simulink model "m02_simulate"  (R2024b)
settings: Solver=VariableStepAuto  StartTime=0.0  StopTime=Tsim  RelTol=1e-3
model workspace (MAT data in the model file):
  C_3 = 1e-07
  Cin_2 = 0.0001
  Cout_2 = 0.0001
  Goff_2 = 1e-06
  L_3 = 0.000277
  L_4 = 0.001
  Len_3 = 1
  Lt_2 = 3.042e-05
  N_2 = 1
  R_1 = 1
  R_3 = 1
  R_c_3 = 1e-06
  Rds_2 = 1e-06
  Rt_2 = 0.001
  Tsim = 0.01
  Tstep = 1e-05
  Vf_2 = 0.001
  fs_2 = 5000
libraries: nesl_utility x7, fl_lib x4, ODEsim x4
settings Model: Creator=cao2851  LastModifiedBy=cao2851
settings DataIOCC: ExternalInput=ds{1}  LoadExternalInput=on

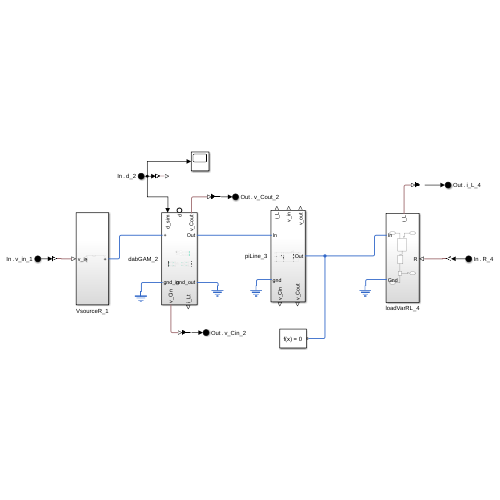
[thumbnail: Simulink's stored preview of the top-level diagram]
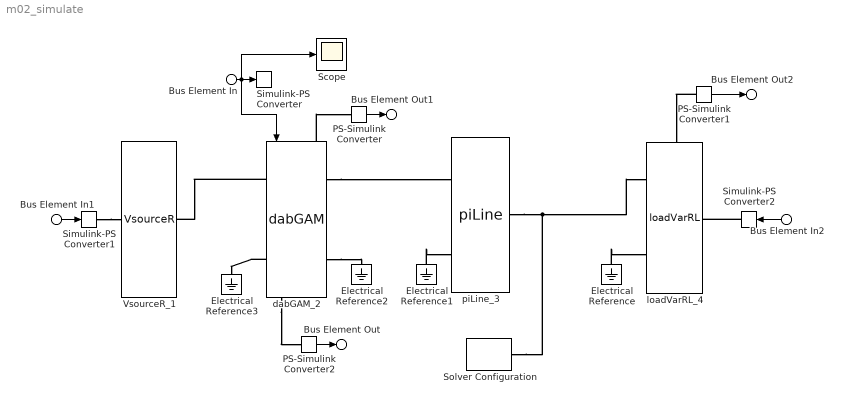
== system m02_simulate ==
  Bus Element In : Inport  PortName=In  Element=d_2
  Bus Element In1 : Inport  PortName=In  Element=v_in_1
  Bus Element In2 : Inport  PortName=In  Element=R_4
  Electrical Reference{,1..3} (4 alike) : fl_lib/Electrical/Electrical Elements/Electrical Reference
  PS-Simulink Converter : nesl_utility/PS-Simulink Converter  PhysicalDomain=network_engine_domain  SubClassName=ps_output  LeftPortType=input  RightPortType=output  PseudoPeriodic=off  Frequencies=[]  VectorFormat=inherit  Unit=inherit  AffineConversion=off
  PS-Simulink Converter1 : nesl_utility/PS-Simulink Converter  PhysicalDomain=network_engine_domain  SubClassName=ps_output  LeftPortType=input  RightPortType=output  PseudoPeriodic=off  Frequencies=[]  VectorFormat=inherit  Unit=inherit  AffineConversion=off
  PS-Simulink Converter2 : nesl_utility/PS-Simulink Converter  PhysicalDomain=network_engine_domain  SubClassName=ps_output  LeftPortType=input  RightPortType=output  PseudoPeriodic=off  Frequencies=[]  VectorFormat=inherit  Unit=inherit  AffineConversion=off
  Scope : Scope
  Simulink-PS Converter : nesl_utility/Simulink-PS Converter  PhysicalDomain=network_engine_domain  SubClassName=ps_input  LeftPortType=input  RightPortType=output  PseudoPeriodic=off  Frequencies=[]  NoiseDistribution=none  NoiseParameters=[]  Unit=1  AffineConversion=off  FilteringAndDerivatives=provide  SimscapeFilterOrder=1  InputFilterTimeConstant=0.001  UdotUserProvided=0
  Simulink-PS Converter1 : nesl_utility/Simulink-PS Converter  PhysicalDomain=network_engine_domain  SubClassName=ps_input  LeftPortType=input  RightPortType=output  PseudoPeriodic=off  Frequencies=[]  NoiseDistribution=none  NoiseParameters=[]  Unit=1  AffineConversion=off  FilteringAndDerivatives=provide  SimscapeFilterOrder=1  InputFilterTimeConstant=0.001  UdotUserProvided=0
  Simulink-PS Converter2 : nesl_utility/Simulink-PS Converter  PhysicalDomain=network_engine_domain  SubClassName=ps_input  LeftPortType=input  RightPortType=output  PseudoPeriodic=off  Frequencies=[]  NoiseDistribution=none  NoiseParameters=[]  Unit=1  AffineConversion=off  FilteringAndDerivatives=provide  SimscapeFilterOrder=1  InputFilterTimeConstant=0.001  UdotUserProvided=0
  Solver Configuration : nesl_utility/Solver Configuration  PhysicalDomain=network_engine_domain  SubClassName=solver  LeftPortType=input  RightPortType=generic  Tones=[]  Harmonics=[]  SimulateNoise=off  Profile=off  UseLocalSampling=off  EnableSwitchedLinearOptims=on  FrequencyDomain=off  UseCCode=off  RelTol=0.001  AbsTol=0.001  MinStep=1e-09  ToWorkspace=off  RevertToSquareIcSolve=off  NumHomotopyIterations=100  PhasorMode=off  PhasorModeNumHarmonics=1  ConsistencySolver=NEWTON_XTOL_AFTER_FTOL  IndexReductionMethod=DerivativeReplacement  DoDC=off  ResidualTolerance=1e-09  ConsistencyTolSource=GLOBAL  ConsistencyAbsTol=0.001  ConsistencyRelTol=0.001  ConsistencyTolFactor=0.001  UseLocalSolver=off  LocalSolverChoice=NE_BACKWARD_EULER_ADVANCER  ResolveIndetEquations=on  FunctionEvalNumThread=1  LocalSolverSampleTime=0.001  DoFixedCost=off  MaxNonlinIter=3  MaxModeIter=2  ComputeImpulses=off  ImpulseIterations=2  LinearAlgebra=auto  LinearAlgebraNumThread=0  EquationFormulation=NE_TIME_EF  DelaysMemoryBudget=1024  AutomaticFiltering=on  FilteringTimeConstant=0.001  PartitionStorageMethod=AS_NEEDED  PartitionMemoryBudget=1024  PartitionMethod=ROBUST  MultibodyUseLocalSolver=off  MultibodyLocalSolverChoice=ODE1  MultibodyLocalSolverSampleTime=0.001
  VsourceR_1 : ODEsim/VsourceR  SystemSampleTime=-1  VariantActivationTime=update diagram  AllowFlexibleInterface=on  Latency=0  AutoFrameSizeCalculation=off
      link override esr: R=R_1
  dabGAM_2 : ODEsim/dabGAM  SystemSampleTime=-1  VariantActivationTime=update diagram  AllowFlexibleInterface=on  Latency=0  AutoFrameSizeCalculation=off
      link override Cin: c=Cin_2
      link override Lt: l=Lt_2  r=Rt_2
      link override S1: Rds=Rds_2  Goff=Goff_2  diode_Goff=Goff_2  diode_Ron=Rds_2  diode_Vf=Vf_2
      link override S2: Rds=Rds_2  Goff=Goff_2  diode_Goff=Goff_2  diode_Ron=Rds_2  diode_Vf=Vf_2
      link override S3: Rds=Rds_2  Goff=Goff_2  diode_Goff=Goff_2  diode_Ron=Rds_2  diode_Vf=Vf_2
      link override S4: Rds=Rds_2  Goff=Goff_2  diode_Goff=Goff_2  diode_Ron=Rds_2  diode_Vf=Vf_2
      link override S5: Rds=Rds_2  Goff=Goff_2  diode_Goff=Goff_2  diode_Ron=Rds_2  diode_Vf=Vf_2
      link override S6: Rds=Rds_2  Goff=Goff_2  diode_Goff=Goff_2  diode_Ron=Rds_2  diode_Vf=Vf_2
      link override S7: Rds=Rds_2  Goff=Goff_2  diode_Goff=Goff_2  diode_Ron=Rds_2  diode_Vf=Vf_2
      link override S8: Rds=Rds_2  Goff=Goff_2  diode_Goff=Goff_2  diode_Ron=Rds_2  diode_Vf=Vf_2
      link override Trf: n=N_2
      link override fs: Value=2*fs_2
      link override fs1: Value=2*fs_2
      settings: PortSchema="{\"entries\":[{\"content\":{\"sides\":[{\"content\":{\"connectorIds\":[\"LConn1\",\"LConn2\"]},\"type\":\"ConnectorPlacement.EquallySpacedRectSide\",\"uuid\":\"349ed430-2934-411c-8d96-d6e1ef881f7a\"},{\"content\":{\"connectorIds\":[\"RConn1\",\"RConn2\"],\"side\":\"RIGHT\"},\"type\":\"ConnectorPlacement.EquallySpacedRectSide\",\"uuid\":\"4c13ef6c-fb55-46d7-8d70-17102cf28db3\"},{\"content\":{\"connectorIds\":[\"In1\",\"LConn3\",\"LConn4\"],\"side\":\"TOP\"},\"type\":\"ConnectorPlacement.EquallySpacedRectSide\",\"uuid\":\"21058841-de4a-4ced-86ff-f9d9fda3a067\"},{\"content\":{\"connectorIds\":[\"RConn3\",\"RConn4\"],\"side\":\"BOTTOM\"},\"type\":\"ConnectorPlacement.EquallySpacedRectSide\",\"uuid\":\"f4d3d5b3-ce7a-4210-8096-b39e7c8d49a1\"}]},\"type\":\"ConnectorPlacement.EquallySpacedConnector\",\"uuid\":\"95c97b55-d26f-4f9a-9092-e1e8cc0ddd5b\"}],\"packageUris\":[\"http://schema.mathworks.com/mf0/Connector/R2020b\"],\"version\":\"1.0\"}"
  loadVarRL_4 : ODEsim/loadVarRL  SystemSampleTime=-1  VariantActivationTime=update diagram  AllowFlexibleInterface=on  Latency=0  AutoFrameSizeCalculation=off
      link override Lload: l=L_4
      settings: PortSchema="{\"entries\":[{\"content\":{\"sides\":[{\"content\":{\"connectorIds\":[\"LConn1\",\"LConn2\"]},\"type\":\"ConnectorPlacement.EquallySpacedRectSide\",\"uuid\":\"3ca054f9-4786-4432-9a42-5c96d58c6caf\"},{\"content\":{\"connectorIds\":[\"RConn1\"],\"side\":\"RIGHT\"},\"type\":\"ConnectorPlacement.EquallySpacedRectSide\",\"uuid\":\"1397a3ce-84de-411a-aceb-8aee73f533ab\"},{\"content\":{\"connectorIds\":[\"LConn3\"],\"side\":\"TOP\"},\"type\":\"ConnectorPlacement.EquallySpacedRectSide\",\"uuid\":\"c1691131-c796-4682-a710-f7ff2056eb7f\"}]},\"type\":\"ConnectorPlacement.EquallySpacedConnector\",\"uuid\":\"16878cab-0730-41de-a010-5d1cfaa9f629\"}],\"packageUris\":[\"http://schema.mathworks.com/mf0/Connector/R2020b\"],\"version\":\"1.0\"}"
  piLine_3 : ODEsim/piLine  SystemSampleTime=-1  VariantActivationTime=update diagram  AllowFlexibleInterface=on  Latency=0  AutoFrameSizeCalculation=off
      link override Cline1: c=C_3 / 2 * Len_3
      link override Cline1_r: R=R_c_3
      link override Cline2: c=C_3 / 2 * Len_3
      link override Cline2_r: R=R_c_3
      link override Lline: l=L_3 * Len_3
      link override Rline: R=R_3 * Len_3
      settings: PortSchema="{\"entries\":[{\"content\":{\"sides\":[{\"content\":{\"connectorIds\":[\"LConn1\",\"LConn2\"]},\"type\":\"ConnectorPlacement.EquallySpacedRectSide\",\"uuid\":\"2f581a64-5488-4115-8fb4-4c7dc7f7cc02\"},{\"content\":{\"connectorIds\":[\"RConn1\"],\"side\":\"RIGHT\"},\"type\":\"ConnectorPlacement.EquallySpacedRectSide\",\"uuid\":\"41fc3ed1-c08d-4cec-81c4-9e5ea37f4b50\"},{\"content\":{\"connectorIds\":[\"LConn3\",\"LConn4\",\"LConn5\"],\"side\":\"TOP\"},\"type\":\"ConnectorPlacement.EquallySpacedRectSide\",\"uuid\":\"f632da0e-7244-44f2-8232-d25344579225\"},{\"content\":{\"connectorIds\":[\"RConn2\",\"RConn3\"],\"side\":\"BOTTOM\"},\"type\":\"ConnectorPlacement.EquallySpacedRectSide\",\"uuid\":\"4895b748-0fce-4270-baa5-001cc2b4bab4\"}]},\"type\":\"ConnectorPlacement.EquallySpacedConnector\",\"uuid\":\"08f1579d-6e1b-4490-ba48-7710ed18f2cd\"}],\"packageUris\":[\"http://schema.mathworks.com/mf0/Connector/R2020b\"],\"version\":\"1.0\"}"
  Bus Element Out : Outport  PortName=Out  Element=v_Cin_2
  Bus Element Out1 : Outport  PortName=Out  Element=v_Cout_2
  Bus Element Out2 : Outport  PortName=Out  Element=i_L_4
  wires:
  PS-Simulink Converter/1 -> Bus Element Out1/1
  PS-Simulink Converter2/1 -> Bus Element Out/1
  PS-Simulink Converter1/1 -> Bus Element Out2/1
  Bus Element In1/1 -> Simulink-PS Converter1/1
  Bus Element In2/1 -> Simulink-PS Converter2/1
  Bus Element In/1 -> dabGAM_2/1, Scope/1, Simulink-PS Converter/1
  connections:
  Electrical Reference/LConn1 -- loadVarRL_4/LConn2
  Electrical Reference1/LConn1 -- piLine_3/LConn2
  piLine_3/RConn1 -- Solver Configuration/RConn1 -- loadVarRL_4/LConn1
  dabGAM_2/RConn1 -- piLine_3/LConn1
  dabGAM_2/RConn2 -- Electrical Reference2/LConn1
  dabGAM_2/LConn2 -- Electrical Reference3/LConn1
  dabGAM_2/LConn4 -- PS-Simulink Converter/LConn1
  PS-Simulink Converter1/LConn1 -- loadVarRL_4/LConn3
  dabGAM_2/RConn3 -- PS-Simulink Converter2/LConn1
  dabGAM_2/LConn1 -- VsourceR_1/RConn1
  Simulink-PS Converter1/RConn1 -- VsourceR_1/LConn1
  Simulink-PS Converter2/RConn1 -- loadVarRL_4/RConn1
